simulink model "model"  (R2020b)
settings: Solver=VariableStepAuto  StartTime=0.0  StopTime=1  FixedStep=Ts  RelTol=1e-3
undefined symbols (not defined in the file): b, J, Ke, Kt, L, R
settings Model: DataDictionary=Motor_position_data.sldd  OrderedModelArguments=off  Creator=Lenovo  LastModifiedBy=Akshata Ashok
settings DataIOCC: SaveOutput=off  SaveTime=off  ReturnWorkspaceOutputs=off

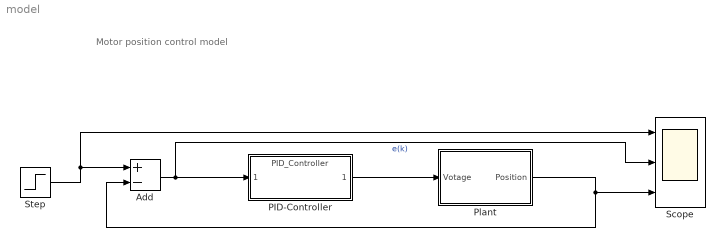
== system model ==
  note: Motor position control model
  Add : Sum  Inputs=+-
  PID-Controller : ModelReference  ModelNameDialog=PID_Controller  SimulationMode=Normal  ModelReferenceVersion=1.51  mask{Kp=18842.98, Ki=12396450.71, Kd=6.98}
  Plant : Subsystem
  Scope : Scope  NumInputPorts=3
  Step : Step  Time=0  SampleTime=0
  wires:
  Plant/1(Position) -> Add/2, Scope/3
  Step/1 -> Add/1, Scope/1
  Add/1 -> PID-Controller/1, Scope/2  "e(k)"
  PID-Controller/1 -> Plant/1(Votage)

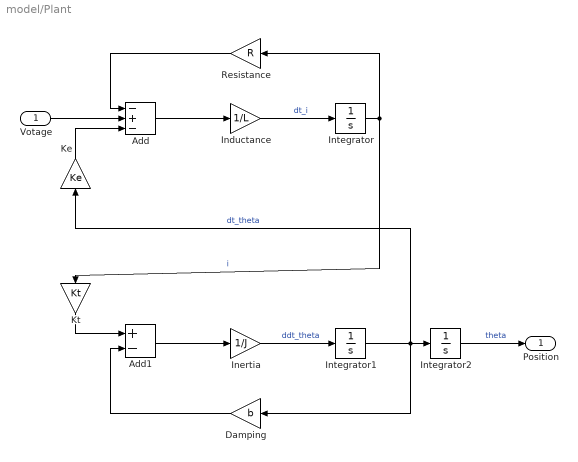
== system model/Plant ==
  Votage : Inport
  Add : Sum  Inputs=-+-
  Add1 : Sum  Inputs=+-
  Damping : Gain  Gain=b
  Inductance : Gain  Gain=1/L
  Inertia : Gain  Gain=1/J
  Integrator : Integrator
  Integrator1 : Integrator
  Integrator2 : Integrator
  Ke : Gain  Gain=Ke
  Kt : Gain  Gain=Kt
  Resistance : Gain  Gain=R
  Position : Outport
  wires:
  Add/1 -> Inductance/1
  Inductance/1 -> Integrator/1  "dt_i"
  Integrator/1 -> Resistance/1, Kt/1  "i"
  Resistance/1 -> Add/1
  Add1/1 -> Inertia/1
  Inertia/1 -> Integrator1/1  "ddt_theta"
  Integrator1/1 -> Ke/1, Integrator2/1, Damping/1  "dt_theta"
  Damping/1 -> Add1/2
  Ke/1 -> Add/3
  Votage/1 -> Add/2
  Kt/1 -> Add1/1
  Integrator2/1 -> Position/1  "theta"
